simulink model "Depth_controller_test"  (R2018a)
settings: Solver=VariableStepAuto  StartTime=0.0  StopTime=500  RelTol=1e-3
settings Model: Creator=梁鑫  LastModifiedBy=梁鑫

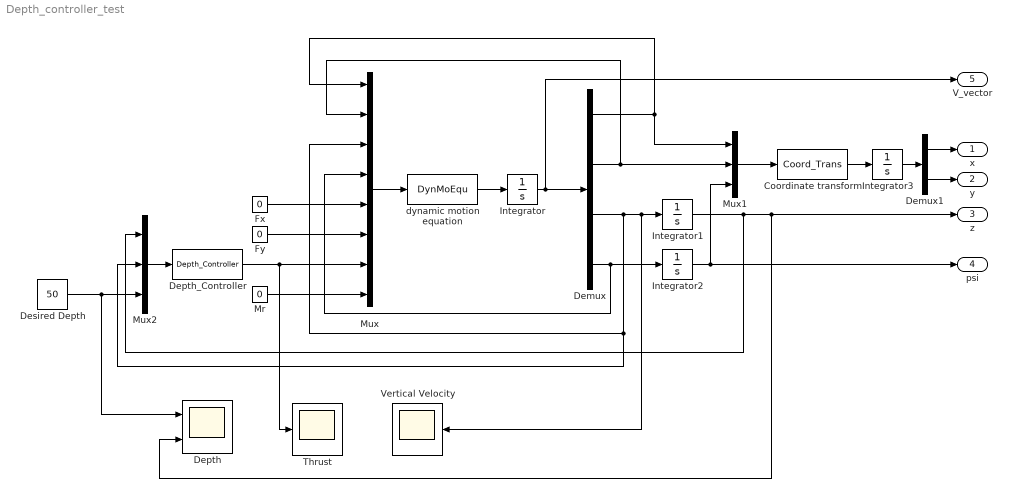
== system Depth_controller_test ==
  Coordinate transform : MATLABFcn  MATLABFcn=Coord_Trans  OutputDimensions=2
  Demux : Demux
  Demux1 : Demux  Outputs=2
  Depth : Scope  NumInputPorts=2
  Depth_Controller : MATLABFcn  MATLABFcn=Depth_Controller  OutputDimensions=1
  Desired Depth : Constant  Value=50
  Fx : Constant  Value=0
  Fy : Constant  Value=0
  Integrator{,1..3} (4 alike) : Integrator
  Mr : Constant  Value=0
  Mux : Mux  Inputs=8
  Mux1 : Mux  Inputs=3
  Mux2 : Mux  Inputs=3
  Thrust : Scope
  Vertical Velocity : Scope
  dynamic motion equation : MATLABFcn  MATLABFcn=DynMoEqu  OutputDimensions=4
  x : Outport
  y : Outport  Port=2
  z : Outport  Port=3
  psi : Outport  Port=4
  V_vector : Outport  Port=5
  wires:
  Integrator1/1 -> Mux2/1, Depth/2, z/1
  Mux/1 -> dynamic motion equation/1
  Integrator3/1 -> Demux1/1
  Coordinate transform/1 -> Integrator3/1
  Demux1/1 -> x/1
  Fx/1 -> Mux/5
  Demux/2 -> Mux/2, Mux1/2
  Mux1/1 -> Coordinate transform/1
  dynamic motion equation/1 -> Integrator/1
  Demux/3 -> Mux2/2, Mux/3, Vertical Velocity/1, Integrator1/1
  Demux/1 -> Mux1/1, Mux/1
  Demux1/2 -> y/1
  Integrator2/1 -> Mux1/3, psi/1
  Demux/4 -> Mux/4, Integrator2/1
  Mr/1 -> Mux/8
  Integrator/1 -> Demux/1, V_vector/1
  Fy/1 -> Mux/6
  Mux2/1 -> Depth_Controller/1
  Depth_Controller/1 -> Thrust/1, Mux/7
  Desired Depth/1 -> Depth/1, Mux2/3
